simulink model "Q1GustavoSim"  (R2022a)
settings: Solver=VariableStepAuto  StartTime=0.0  StopTime=10.0  RelTol=1e-3
values from neighbouring files (symbols this model uses):
  K1 = acker(A,B,P1)    [Q1Gustavo.m]
settings Model: Creator=gusta  LastModifiedBy=gusta

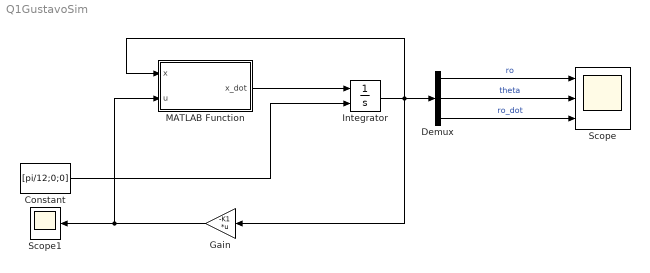
== system Q1GustavoSim ==
  Constant : Constant  Value=[pi/12;0;0]  VectorParams1D=off
  Demux : Demux  Outputs=3
  Gain : Gain  Gain=-K1  Multiplication=Matrix(K*u)
  Integrator : Integrator  InitialConditionSource=external
  MATLAB Function : MATLAB Function  TreatAsAtomicUnit=on
  Scope : Scope  NumInputPorts=3
  Scope1 : Scope
  wires:
  MATLAB Function/1(x_dot) -> Integrator/1
  Integrator/1 -> Gain/1, Demux/1, MATLAB Function/1(x)
  Constant/1 -> Integrator/2
  Gain/1 -> MATLAB Function/2(u), Scope1/1
  Demux/1 -> Scope/1  "ro"
  Demux/2 -> Scope/2  "theta"
  Demux/3 -> Scope/3  "ro_dot"

== matlab function Q1GustavoSim/MATLAB Function ==
  data: x input; u input; x_dot output
function x_dot = gyro_model(x,u)
    %x1 = ro; x2=theta; x3=ro_dot; u=theta_dot;

    mV = .430; % [kg] massa do veículo, excluindo giroscópio e objeto
    mG = .190; % [kg] massa do giroscópio
    rG = 2*.05; % [m] raio do giroscópio
    aG = -1*.02; % [m] distância entre o centro de massa do giroscópio e ponto de rotação
    aV = .1; % [m] altura do veículo
    lV = .035; % [m] largura do veículo
    dG = .1+.02;
    dV = .1;
    omega = 3000*10472; % rpm * conversion factor = rad/sec
    g = 9.81; % [m/s^2] aceleração da gravidade
    IG11 = (mG*(rG^2)/4) + (mG*(dG^2)/12); % IG22 = IG11
    IG33 = (mG*(rG^2))/2;
    IB11 = mV*((aV^2)+(lV^2))/12;
    
    x1 = x(1);
    x2 = x(2);
    x3 = x(3);
    
    f1 = x3;
    f2 = 0;
    f3 = ((mV*dV+mG*dG)*g*sin(x1))/((IB11+mV*(dV^2)+IG11*((cos(x2))^2))+mG*(dG^2)+IG33*((sin(x2))^2));
    g1 = 0;
    g2 = 1;
    g3 = ((-2*cos(x2)*sin(x2)*x3*(IG33-IG11)-omega*cos(x2)*IG33))/((IB11+IG11*(cos(x2)^2)+mV*(dV^2)+mG*(dG^2)));

    f = [f1;f2;f3];
    g = [g1;g2;g3];

    x_dot = f + g*u;
end
